simulink model "ExoskeletonControlModel"  (R2022b)
settings: Solver=ode3  StartTime=0.0  StopTime=inf  FixedStep=Ts  RelTol=1e-3
PreLoadFcn:
  | Ts_IO204 = 0.001;
  | 
  | if ~exist('Ts', 'var')
  | Ts = 0.001;
  | end
  | if ~exist('FPGA_Frequency', 'var')
  | FPGA_Frequency = 75000000;
  | end
  | 
  | ts_IO612 = 1e-3;
  | 
  | load('TargetReached.mat')
  | load('ActualPos_inc.mat')
model workspace (MAT data in the model file):
  DeltaData : timeseries (value not decoded)
  EC45_deg2incs = 2276
  EC60_deg2inc = 5461
  EC90_deg2incs = 7111
  Enc2rad_18bit = 2.3968e-05
  Enc2rad_19bit = 1.1984e-05
  Enc2rad_20bit = 5.9921e-06
  GiulioModel : robotics.RigidBodyTree (value not decoded)
  Giulio_Spheric_model : robotics.RigidBodyTree (value not decoded)
  Offset1_ticks = 571315
  Offset2_ticks = 590938.9928
  Offset3_ticks = 457912.8279
  Offset4_ticks = 482293.9763
  Offset5_ticks = 598735.9316
  Offset_M1 = 1.12645499896
  Offset_M2 = 4.02728553608
  Offset_M3 = 5.48587511336
  Offset_M4 = 2.03717511516
  Offset_M5 = 4.4996674016
  T1_Nm : object (value not decoded)
  T2_Nm : object (value not decoded)
  TBmodel : robotics.RigidBodyTree (value not decoded)
  Ts = 0.002
  Xg : object (value not decoded)
  Yg : object (value not decoded)
  Zg : object (value not decoded)
  a2 = 0.27
  change_variable = 0
  d1 = [0 0 0 0 0 0 0 0 0 0 0 0 ... (30001 elements, 30001x1)]
  d1_1 = 0.21074
  d2 = [0 0 0 0 0 0 0 0 0 0 0 0 ... (30001 elements, 30001x1)]
  d2_1 = 0.04864
  d3 = [0 0 0 0 0 0 0 0 0 0 0 0 ... (30001 elements, 30001x1)]
  d4 = [0 0 0 0 0 0 0 0 0 0 0 0 ... (30001 elements, 30001x1)]
  d5 = [0 0 0 0 0 0 0 0 0 0 0 0 ... (30001 elements, 30001x1)]
  d6 = [0 0 0 0 0 0 0 0 0 0 0 0 ... (30001 elements, 30001x1)]
  ee_x = -0.2852
  ee_y = -0.3683
  ee_z = -0.0386
  enc2rad_EC45 = 7.6699e-06
  enc2rad_EC90 = 2.3969e-05
  k1_Nm_ticks = 0.00923
  k2_Nm_ticks = 0.0257
  k3_Nm_ticks = 0.00692
  k4_Nm_ticks = 0.00729
  k5_Nm_ticks = 0.00641
  lower_lim_m1 = -330000
  lower_lim_m2 = -235302
  lower_lim_m3 = -132865
  lower_lim_m4 = -152732
  lower_lim_m5 = -138363
  lower_lim_m6 = -200325
  m1 = 2.441408578
  m2 = 3.750007
  m3 = 1.56250298
  m4 = 1.56250298
  m5 = 1.56250298
  m6 = 1.56250298
  n_oversampling = 8
  offset_sea_1 = 0.5547
  offset_sea_2 = 2.8595
  offset_sea_3 = 3.5058
  offset_sea_4 = 2.8586
  offset_sea_5 = 2.8736
  params : AKSIM (value not decoded)
  pos_th_neg = -180000
  pos_th_pos = 180000
  q1 = -1819347
  q2 = -196752
  q3 = -596465
  q4 = -556807
  q5 = -573932
  q6 = -489063
  sine = [0 0.187999937334 0.751998997352 1.69199492401 3.0079839574 4.6999608335 6.76791878442 9.21184953835 12.0317433196 15.2275888485 18.7993733417 22.7470825122 ... (12501 elements, 12501x1)]
  start : object (value not decoded)
  switch_admittance = 1
  t1 : object (value not decoded)
  t2 : object (value not decoded)
  torsionalStiffnes_M1 = 384.88
  torsionalStiffnes_M2 = 1500
  torsionalStiffnes_M3 = 901.97
  torsionalStiffnes_M4 = 950.86
  torsionalStiffnes_M5 = 930
  torsionalStiffnes_M6 = 914
  upper_lim_m1 = 340000
  upper_lim_m2 = 95467
  upper_lim_m3 = 164951
  upper_lim_m4 = 210607
  upper_lim_m5 = 252595
  upper_lim_m6 = 96694
  vel_th_neg = -100
  vel_th_pos = 100
  x = 0
undefined symbols (not defined in the file): C, DiscIntNeverNeededParam
libraries: canmsglib x285, speedgoatlib_IO614 x245, simulink x26, slrealtimeloglib x9, simulink_extras x6, robotmaniplib x6
(part 9 of 13)

== system ExoskeletonControlModel/OutputDataTX/TX_EPOS4_M3_M5/rxSDO4 ==
  Trigger : TriggerPort  VariantControl=Variant  PortDimensions=1
  CAN Write : speedgoatlib_IO614/CAN/CAN Write  id=1  sampleTime=-1  portSelection=4  messageType=CAN  enaStatusPort=off  protl=IO614  ptIdx=3  isFDMod=0
  CS : Constant  Value=hex2dec('40')
  Index : Constant  Value=hex2dec('3012')
  ParamData : Constant  Value=hex2dec('000F')
  Subindex : Constant  Value=hex2dec('09')
  rxSDO : canmsglib/CAN Pack  MsgList=(none)  MsgName=CAN Msg  MsgIDType=Standard (11-bit identifier)  MsgIdentifier=1540  MsgLength=8  Remote=off  ApplyMinMax=off  BusOutput=off  SignalInfo={ 'CS', '0', '8', 'LE', 'unsigned', 'Standard', '0', '1', '0', '-Inf', 'Inf'; 'Index', '8', '16', 'LE', 'unsigned', 'Standard', '0', '1', '0', '-Inf', 'Inf'; 'SubIndex', '24', '8', 'LE', 'unsigned', 'Standard', '0', '1', '0', '-Inf', 'Inf'; 'ParamData', '32', '32', 'LE', 'signed', 'Standard', '0', '1', '0', '-Inf', 'Inf' }
      settings: DataFormat=manually specified signals
  wires:
  rxSDO/1 -> CAN Write/1
  CS/1 -> rxSDO/1
  Index/1 -> rxSDO/2
  Subindex/1 -> rxSDO/3
  ParamData/1 -> rxSDO/4

== system ExoskeletonControlModel/OutputDataTX/TX_EPOS4_M3_M5/set_NMT_state ==
  Input : Inport
  Trigger : TriggerPort  VariantControl=Variant  PortDimensions=1
  CAN Write : speedgoatlib_IO614/CAN/CAN Write  id=1  sampleTime=-1  portSelection=4  messageType=CAN  enaStatusPort=off  protl=IO614  ptIdx=3  isFDMod=0
  NodeID : Constant  Value=0
  set_NMT_state : canmsglib/CAN Pack  MsgList=(none)  MsgName=CAN Msg  MsgIDType=Standard (11-bit identifier)  MsgIdentifier=0  MsgLength=2  Remote=off  ApplyMinMax=off  BusOutput=off  SignalInfo={ 'CS', '0', '8', 'LE', 'unsigned', 'Standard', '0', '1', '0', '-Inf', 'Inf'; 'NodeID', '8', '8', 'LE', 'unsigned', 'Standard', '0', '1', '0', '-Inf', 'Inf' }
      settings: DataFormat=manually specified signals
  wires:
  Input/1 -> set_NMT_state/1
  NodeID/1 -> set_NMT_state/2
  set_NMT_state/1 -> CAN Write/1

== system ExoskeletonControlModel/DataProcessing/CST_trasparency/CST_control/MOTOR3 ==
  note: FrictionCompensation
  note: IMPEDENCE CONTROL M3
  note: CURRENT CONTROL M3
  TauSEA : Inport
  Gravity : Inport  Port=2
  position : Inport  Port=3
  speed_rads : Inport  Port=4
  State : Inport  Port=5
  MovLenght : Inport  Port=6
  Reset : Inport  Port=7
  Enable : EnablePort
  Abs : Abs  SaturateOnIntegerOverflow=off
  Chart : Stateflow chart  TreatAsAtomicUnit=on
  Constant1 : Constant  Value=-0.1
  Data Store Read : DataStoreRead  DataStoreName=Start_m3  IndexOptions=Index vector (dialog)  Indices=1  OutputSizes=1
  Data Store Read2 : DataStoreRead  DataStoreName=Spring_m3  IndexOptions=Index vector (dialog)  Indices=1  OutputSizes=1
  Degrees to Radians : simulink_extras/Transformations/Degrees to Radians
  Delay1 : Delay  DelayLength=1
  Enc2rad : Gain  Gain=1/(2276)
  Gain : Gain  Gain=1/100
  Gain1 : Gain  Gain=9.5492965964254
  Product : Product
  Product2 : Product
  Product3 : Product
  Subsystem1 : Subsystem
  Sum : Sum  Inputs=|++
  Sum2 : Sum  Inputs=|-+
  Sum3 : Sum  Inputs=|++
  Sum4 : Sum  Inputs=|+-
  Sum5 : Sum  Inputs=++++
  Terminator : Terminator
  Terminator1 : Terminator
  Thousands of nominal torque EC2 : Gain  Gain=8442.5
  impedance_values_safe_zones : Stateflow chart  TreatAsAtomicUnit=on
  Reference Drive Current | Volt1 : Outport
  SignalEnded3 : Outport  Port=2  InitialOutput=0
  LeR_M3 : Outport  Port=3  InitialOutput=0
  wires:
  Sum5/1 -> Product/2
  Enc2rad/1 -> Degrees to Radians/1  "DeltaPos_rad"
  Sum4/1 -> Enc2rad/1  "DeltaPos_inc"
  impedance_values_safe_zones/1(new_target_torque) -> Sum5/3
  Subsystem1/1(RefPosLR) -> LeR_M3/1, Sum4/1
  Gravity/1 -> Sum/2, Sum5/1
  impedance_values_safe_zones/2(y) -> Terminator1/1
  Sum3/1 -> Sum/1, impedance_values_safe_zones/1(torque)
  Constant1/1 -> Sum3/2
  Degrees to Radians/1 -> Product2/1
  TauSEA/1 -> Sum3/1
  Data Store Read2/1 -> Product2/2
  Data Store Read/1 -> Product/1
  position/1 -> impedance_values_safe_zones/2(theta), Sum4/2
  Product/1 -> Thousands of nominal torque EC2/1
  Thousands of nominal torque EC2/1 -> Gain/1  "Reference Drive Current | Volt"
  Sum/1 -> Sum5/2
  Gain/1 -> Reference Drive Current | Volt1/1
  speed_rads/1 -> Gain1/1, Product3/2, impedance_values_safe_zones/3(speed)
  Chart/1(beta) -> Product3/1
  Abs/1 -> Chart/2(speed)
  State/1 -> Chart/1(state)
  Gain1/1 -> Abs/1
  Sum2/1 -> Sum5/4
  Product3/1 -> Sum2/1
  MovLenght/1 -> Subsystem1/2(sz)
  Reset/1 -> Subsystem1/Enable, Delay1/1
  Delay1/1 -> Subsystem1/1(In1)
  Subsystem1/3(Out2) -> Terminator/1
  Subsystem1/2(signal_ended) -> SignalEnded3/1
  Product2/1 -> Sum2/2

== system ExoskeletonControlModel/DataProcessing/CST_trasparency/CST_control/MOTOR4 ==
  note: CURRENT CONTROL M4
  note: IMPEDENCE CONTROL M4
  note: FrictionCompensation
  TauSEA : Inport
  Gravity : Inport  Port=2
  position : Inport  Port=3
  speed_rads : Inport  Port=4
  In6 : Inport  Port=5
  MovLenght : Inport  Port=6
  Reset : Inport  Port=7
  Enable : EnablePort
  Abs : Abs  SaturateOnIntegerOverflow=off
  Chart : Stateflow chart  TreatAsAtomicUnit=on
  Constant : Constant  Value=-0.1
  Data Store Read : DataStoreRead  DataStoreName=Start_m4  IndexOptions=Index vector (dialog)  Indices=1  OutputSizes=1
  Data Store Read2 : DataStoreRead  DataStoreName=Spring_m4  IndexOptions=Index vector (dialog)  Indices=1  OutputSizes=1
  Degrees to Radians : simulink_extras/Transformations/Degrees to Radians
  Delay1 : Delay  DelayLength=1
  Enc2rad : Gain  Gain=1/(2276)
  Gain : Gain  Gain=1/100
  Gain1 : Gain  Gain=9.5492965964254
  Product : Product
  Product2 : Product
  Product3 : Product
  Subsystem1 : Subsystem
  Sum : Sum  Inputs=|++
  Sum2 : Sum  Inputs=|++
  Sum3 : Sum  Inputs=|+-
  Sum4 : Sum  Inputs=++++
  Sum5 : Sum  Inputs=|-+
  Terminator : Terminator
  Terminator1 : Terminator
  Thousands of nominal torque EC2 : Gain  Gain=8442.5
  impedance_values_safe_zones : Stateflow chart  TreatAsAtomicUnit=on
  Reference Drive Current | Volt1 : Outport
  SignalEnded3 : Outport  Port=2
  LeR_M4 : Outport  Port=3
  wires:
  Constant/1 -> Sum2/2
  impedance_values_safe_zones/2(y) -> Terminator1/1
  Gravity/1 -> Sum/1, Sum4/1
  position/1 -> impedance_values_safe_zones/2(theta), Sum3/2
  Data Store Read/1 -> Product/1
  impedance_values_safe_zones/1(new_target_torque) -> Sum4/3
  Product2/1 -> Sum5/2
  Sum3/1 -> Enc2rad/1  "DeltaPos_inc"
  Degrees to Radians/1 -> Product2/1
  Subsystem1/1(RefPosLR) -> LeR_M4/1, Sum3/1
  Sum4/1 -> Product/2
  Enc2rad/1 -> Degrees to Radians/1  "DeltaPos_rad"
  TauSEA/1 -> Sum2/1
  Sum2/1 -> Sum/2, impedance_values_safe_zones/1(torque)
  Data Store Read2/1 -> Product2/2
  Product/1 -> Thousands of nominal torque EC2/1
  Thousands of nominal torque EC2/1 -> Gain/1  "Reference Drive Current | Volt"
  Gain/1 -> Reference Drive Current | Volt1/1
  Sum/1 -> Sum4/2
  Chart/1(beta) -> Product3/1
  Gain1/1 -> Abs/1
  speed_rads/1 -> Product3/2, Gain1/1, impedance_values_safe_zones/3(speed)
  Product3/1 -> Sum5/1
  In6/1 -> Chart/1(state)
  Abs/1 -> Chart/2(speed)
  Sum5/1 -> Sum4/4
  Subsystem1/3(Out2) -> Terminator/1
  MovLenght/1 -> Subsystem1/2(sz)
  Delay1/1 -> Subsystem1/1(In1)
  Reset/1 -> Delay1/1, Subsystem1/Enable
  Subsystem1/2(signal_ended) -> SignalEnded3/1

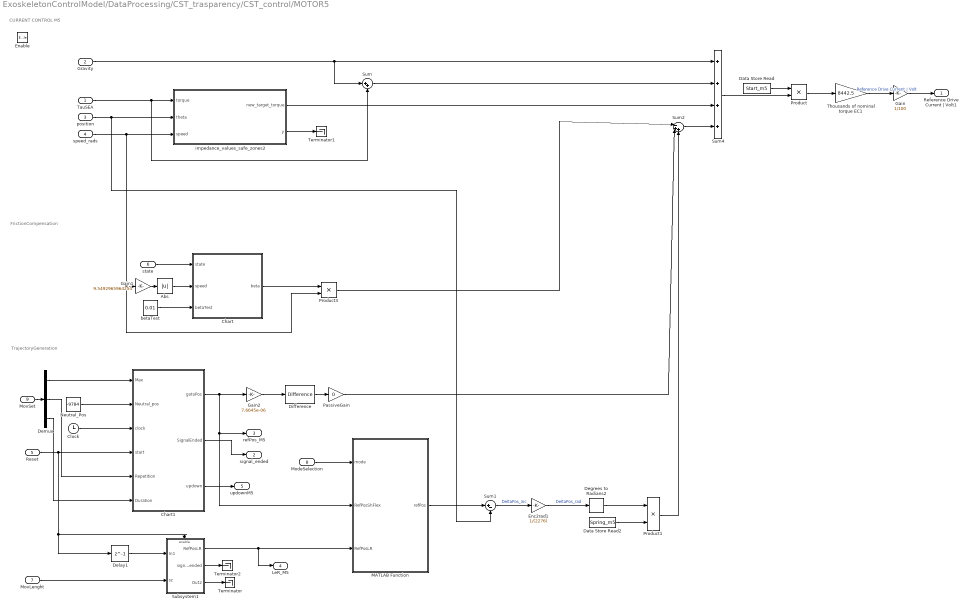
== system ExoskeletonControlModel/DataProcessing/CST_trasparency/CST_control/MOTOR5 ==
  note: TrajectoryGeneration
  note: CURRENT CONTROL M5
  note: FrictionCompensation
  TauSEA : Inport
  Gravity : Inport  Port=2
  position : Inport  Port=3
  speed_rads : Inport  Port=4
  Reset : Inport  Port=5
  state : Inport  Port=6
  MovLenght : Inport  Port=7
  ModeSelection : Inport  Port=8
  MovSet : Inport  Port=9
  Enable : EnablePort
  Abs : Abs  SaturateOnIntegerOverflow=off
  Chart : Stateflow chart  TreatAsAtomicUnit=on
  Chart1 : Stateflow chart  TreatAsAtomicUnit=on
  Clock : Clock
      settings: Decimation=1000
  Data Store Read : DataStoreRead  DataStoreName=Start_m5  IndexOptions=Index vector (dialog)  Indices=1  OutputSizes=1
  Data Store Read2 : DataStoreRead  DataStoreName=Spring_m5  IndexOptions=Index vector (dialog)  Indices=1  OutputSizes=1
  Degrees to Radians2 : simulink_extras/Transformations/Degrees to Radians
  Delay1 : Delay  DelayLength=1
  Demux : Demux  Outputs=3
  Difference : simulink/Discrete/Difference  ICPrevInput=0.0  OutMin=[]  OutMax=[]  OutDataType=fixdt(1, 16)  OutScaling=2^-10  DoSatur=off
  Enc2rad1 : Gain  Gain=1/(2276)
  Gain : Gain  Gain=1/100
  Gain1 : Gain  Gain=9.5492965964254
  Gain2 : Gain  Gain=7.6645e-06
  MATLAB Function : MATLAB Function  TreatAsAtomicUnit=on
  Neutral_Pos : Constant  Value=-9784
  PassiveGain : Gain  Gain=0
  Product : Product
  Product1 : Product
  Product3 : Product
  Subsystem1 : Subsystem
  Sum : Sum  Inputs=|++
  Sum1 : Sum  Inputs=|+-
  Sum2 : Sum  Inputs=|-++
  Sum4 : Sum  Inputs=++++
  Terminator : Terminator
  Terminator1 : Terminator
  Terminator2 : Terminator
  Thousands of nominal torque EC1 : Gain  Gain=8442.5
  betaTest : Constant  Value=0.01
  impedance_values_safe_zones2 : Stateflow chart  TreatAsAtomicUnit=on
  Reference Drive Current | Volt1 : Outport
  signal_ended : Outport  Port=2  InitialOutput=0
  refPos_M5 : Outport  Port=3
  LeR_M5 : Outport  Port=4
  updownM5 : Outport  Port=5  InitialOutput=0
  wires:
  impedance_values_safe_zones2/1(new_target_torque) -> Sum4/3
  Sum4/1 -> Product/2
  Gravity/1 -> Sum/1, Sum4/1
  Thousands of nominal torque EC1/1 -> Gain/1  "Reference Drive Current | Volt"
  TauSEA/1 -> Sum/2, impedance_values_safe_zones2/1(torque)
  impedance_values_safe_zones2/2(y) -> Terminator1/1
  Data Store Read/1 -> Product/1
  Product3/1 -> Sum2/1
  speed_rads/1 -> impedance_values_safe_zones2/3(speed), Gain1/1, Product3/2
  position/1 -> impedance_values_safe_zones2/2(theta), Sum1/2
  Sum2/1 -> Sum4/4
  Sum/1 -> Sum4/2
  Gain/1 -> Reference Drive Current | Volt1/1
  Product/1 -> Thousands of nominal torque EC1/1
  Abs/1 -> Chart/2(speed)
  Gain1/1 -> Abs/1
  state/1 -> Chart/1(state)
  Product1/1 -> Sum2/3
  Neutral_Pos/1 -> Chart1/2(Neutral_pos)
  Chart1/1(gotoPos) -> refPos_M5/1, MATLAB Function/2(RefPosShFlex), Gain2/1
  Clock/1 -> Chart1/3(clock)
  Chart1/2(SignalEnded) -> signal_ended/1
  Data Store Read2/1 -> Product1/2
  Sum1/1 -> Enc2rad1/1  "DeltaPos_inc"
  Enc2rad1/1 -> Degrees to Radians2/1  "DeltaPos_rad"
  Degrees to Radians2/1 -> Product1/1
  Gain2/1 -> Difference/1
  Difference/1 -> PassiveGain/1
  PassiveGain/1 -> Sum2/2
  Delay1/1 -> Subsystem1/1(In1)
  MovLenght/1 -> Subsystem1/2(sz)
  Reset/1 -> Subsystem1/Enable, Delay1/1, Chart1/4(start)
  ModeSelection/1 -> MATLAB Function/1(mode)
  MATLAB Function/1(refPos) -> Sum1/1
  Subsystem1/1(RefPosLR) -> LeR_M5/1, MATLAB Function/3(RefPosLR)
  Subsystem1/3(Out2) -> Terminator/1
  Subsystem1/2(signal_ended) -> Terminator2/1
  Chart/1(beta) -> Product3/1
  betaTest/1 -> Chart/3(betaTest)
  Chart1/3(updown) -> updownM5/1
  Demux/1 -> Chart1/1(Max)
  Demux/2 -> Chart1/5(Repetition)
  Demux/3 -> Chart1/6(Duration)
  MovSet/1 -> Demux/1

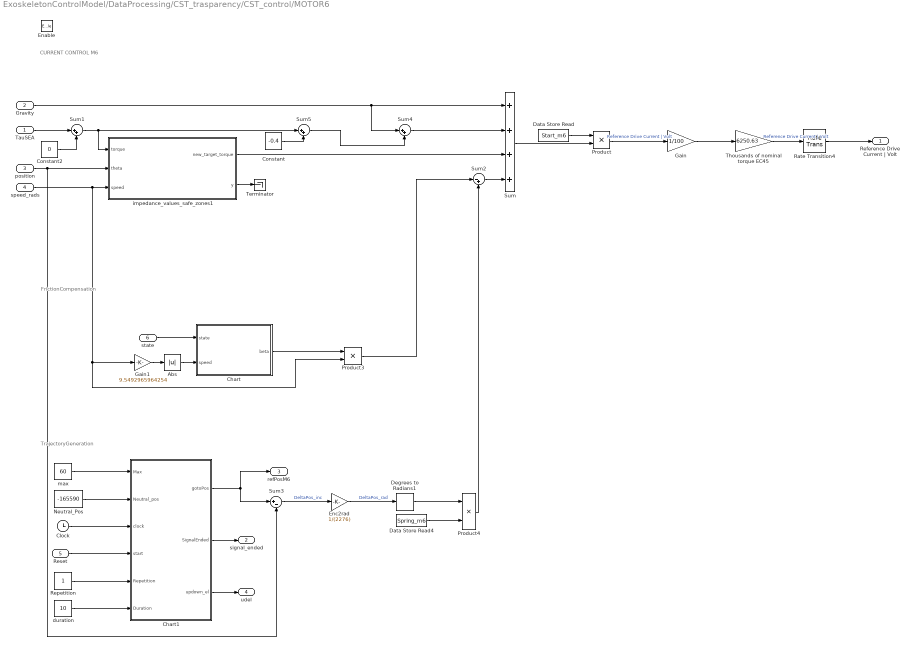
== system ExoskeletonControlModel/DataProcessing/CST_trasparency/CST_control/MOTOR6 ==
  note: TrajectoryGeneration
  note: CURRENT CONTROL M6
  note: FrictionCompensation
  TauSEA : Inport
  Gravity : Inport  Port=2
  position : Inport  Port=3
  speed_rads : Inport  Port=4
  Reset : Inport  Port=5
  state : Inport  Port=6
  Enable : EnablePort
  Abs : Abs  SaturateOnIntegerOverflow=off
  Chart : Stateflow chart  TreatAsAtomicUnit=on
  Chart1 : Stateflow chart  TreatAsAtomicUnit=on
  Clock : Clock
      settings: Decimation=1000
  Constant : Constant  Value=-0.4
  Constant2 : Constant  Value=0
  Data Store Read : DataStoreRead  DataStoreName=Start_m6  IndexOptions=Index vector (dialog)  Indices=1  OutputSizes=1
  Data Store Read4 : DataStoreRead  DataStoreName=Spring_m6  IndexOptions=Index vector (dialog)  Indices=1  OutputSizes=1
  Degrees to Radians1 : simulink_extras/Transformations/Degrees to Radians
  Enc2rad : Gain  Gain=1/(2276)
  Gain : Gain  Gain=1/100
  Gain1 : Gain  Gain=9.5492965964254
  Neutral_Pos : Constant  Value=-165590
  Product : Product
  Product3 : Product
  Product4 : Product
  Rate Transition4 : RateTransition  Deterministic=off  OutPortSampleTime=Ts
  Repetition : Constant
  Sum : Sum  Inputs=++++
  Sum1 : Sum  Inputs=|++
  Sum2 : Sum  Inputs=|-+
  Sum3 : Sum  Inputs=|+-
  Sum4 : Sum  Inputs=|++
  Sum5 : Sum  Inputs=|++
  Terminator : Terminator
  Thousands of nominal torque EC45 : Gain  Gain=6250.63
  duration : Constant  Value=10
  impedance_values_safe_zones1 : Stateflow chart  TreatAsAtomicUnit=on
  max : Constant  Value=60
  Reference Drive Current | Volt : Outport
  signal_ended : Outport  Port=2  InitialOutput=0
  refPosM6 : Outport  Port=3
  udel : Outport  Port=4  InitialOutput=0
  wires:
  Sum/1 -> Product/2
  impedance_values_safe_zones1/1(new_target_torque) -> Sum/3
  Reset/1 -> Chart1/4(start)
  impedance_values_safe_zones1/2(y) -> Terminator/1
  Data Store Read/1 -> Product/1
  speed_rads/1 -> Product3/2, Gain1/1, impedance_values_safe_zones1/3(speed)
  position/1 -> impedance_values_safe_zones1/2(theta), Sum3/2
  Sum3/1 -> Enc2rad/1  "DeltaPos_inc"
  Sum2/1 -> Sum/4
  Product3/1 -> Sum2/1
  Enc2rad/1 -> Degrees to Radians1/1  "DeltaPos_rad"
  Product4/1 -> Sum2/2
  Data Store Read4/1 -> Product4/2
  Degrees to Radians1/1 -> Product4/1
  Chart/1(beta) -> Product3/1
  Sum1/1 -> Sum5/1, impedance_values_safe_zones1/1(torque)
  TauSEA/1 -> Sum1/1
  Constant2/1 -> Sum1/2
  Rate Transition4/1 -> Reference Drive Current | Volt/1
  Product/1 -> Gain/1  "Reference Drive Current | Volt"
  Gain/1 -> Thousands of nominal torque EC45/1
  Thousands of nominal torque EC45/1 -> Rate Transition4/1  "Reference Drive Current | Volt"
  Gravity/1 -> Sum4/1, Sum/1
  Sum4/1 -> Sum/2
  Constant/1 -> Sum5/2
  Sum5/1 -> Sum4/2
  state/1 -> Chart/1(state)
  Gain1/1 -> Abs/1
  Abs/1 -> Chart/2(speed)
  Repetition/1 -> Chart1/5(Repetition)
  Clock/1 -> Chart1/3(clock)
  Chart1/2(SignalEnded) -> signal_ended/1
  duration/1 -> Chart1/6(Duration)
  Neutral_Pos/1 -> Chart1/2(Neutral_pos)
  max/1 -> Chart1/1(Max)
  Chart1/1(gotoPos) -> Sum3/1, refPosM6/1
  Chart1/3(updown_el) -> udel/1

== system ExoskeletonControlModel/DataProcessing/CST_trasparency/CST_control/SendPositionToEPOS ==
  note: SEND TARGET POSITION TO EPOS SERVOMOTOR CONTROLLER
  PosM5 : Inport
  Enable : EnablePort
  Constant : Constant  Value=-165590
  receive_PDO3_m5 : Subsystem
  receive_PDO3_m6 : Subsystem
  wires:
  PosM5/1 -> receive_PDO3_m5/1(target_pos)  "PositionCommandEPOSM5_inc"
  Constant/1 -> receive_PDO3_m6/1(target_pos)  "PositionCommandEPOSM6_inc"

== system ExoskeletonControlModel/DataProcessing/CST_trasparency/CST_control/SendPositionToEPOS1 ==
  note: SEND TARGET POSITION TO EPOS SERVOMOTOR CONTROLLER
  PosM6 : Inport
  Enable : EnablePort
  Constant : Constant  Value=-9784
  receive_PDO3_m5 : Subsystem
  receive_PDO3_m6 : Subsystem
  wires:
  Constant/1 -> receive_PDO3_m5/1(target_pos)  "PositionCommandEPOSM5_inc"
  PosM6/1 -> receive_PDO3_m6/1(target_pos)  "PositionCommandEPOSM6_inc"

== system ExoskeletonControlModel/DataProcessing/CST_trasparency/CST_control/SendPositionToEPOS2 ==
  note: SEND TARGET POSITION TO EPOS SERVOMOTOR CONTROLLER
  PosM3 : Inport
  PosM4 : Inport  Port=2
  PosM5 : Inport  Port=3
  Enable : EnablePort
  receive_PDO3_m1 : Subsystem
  receive_PDO3_m5 : Subsystem
  receive_PDO3_m6 : Subsystem
  wires:
  PosM5/1 -> receive_PDO3_m5/1(target_pos)  "PositionCommandEPOSM5_inc"
  PosM3/1 -> receive_PDO3_m6/1(target_pos)  "PositionCommandEPOSM6_inc"
  PosM4/1 -> receive_PDO3_m1/1(target_pos)  "PositionCommandEPOSM5_inc"

== system ExoskeletonControlModel/DataProcessing/CST_trasparency/SendTorqueCommand/Subsystem ==
  TAU_M6 : Inport
  Enable : EnablePort
  Bus Creator7 : BusCreator  Inputs=3
  receive_PDO4_m6 : Subsystem
  target_velocity_m6 : Constant  Value=0  SampleTime=-1
  torque_offset_m6 : Constant  Value=0  SampleTime=-1
  wires:
  torque_offset_m6/1 -> Bus Creator7/3  "torque_offset_m6"
  TAU_M6/1 -> Bus Creator7/2
  target_velocity_m6/1 -> Bus Creator7/1  "target_velocity_m6"
  Bus Creator7/1 -> receive_PDO4_m6/1(velocity_torque_offset)

== system ExoskeletonControlModel/DataProcessing/CST_trasparency/SendTorqueCommand/Subsystem1 ==
  TAU_M4 : Inport
  Enable : EnablePort
  Bus Creator1 : BusCreator  Inputs=3
  receive_PDO4_m4 : Subsystem
  target_velocity_m4 : Constant  Value=0
  torque_offset_m4 : Constant  Value=0
  wires:
  Bus Creator1/1 -> receive_PDO4_m4/1(velocity_torque_offset)
  torque_offset_m4/1 -> Bus Creator1/3  "torque_offset_m4"
  target_velocity_m4/1 -> Bus Creator1/1  "target_velocity_m4"
  TAU_M4/1 -> Bus Creator1/2

== system ExoskeletonControlModel/DataProcessing/CST_trasparency/SendTorqueCommand/Subsystem2 ==
  TAU_M5 : Inport
  Enable : EnablePort
  Bus Creator2 : BusCreator  Inputs=3
  receive_PDO4_m5 : Subsystem
  target_velocity_m5 : Constant  Value=0
  torque_offset_m5 : Constant  Value=0
  wires:
  TAU_M5/1 -> Bus Creator2/2
  target_velocity_m5/1 -> Bus Creator2/1  "target_velocity_m5"
  Bus Creator2/1 -> receive_PDO4_m5/1(velocity_torque_offset)
  torque_offset_m5/1 -> Bus Creator2/3  "torque_offset_m5"

== system ExoskeletonControlModel/DataProcessing/CST_trasparency/SendTorqueCommand/Subsystem3 ==
  TAU_M3 : Inport
  Enable : EnablePort
  Bus Creator : BusCreator  Inputs=3
  receive_PDO4_m3 : Subsystem
  target_velocity_m3 : Constant  Value=0
  torque_offset_m3 : Constant  Value=0
  wires:
  TAU_M3/1 -> Bus Creator/2
  Bus Creator/1 -> receive_PDO4_m3/1(velocity_torque_offset)
  target_velocity_m3/1 -> Bus Creator/1  "target_velocity_m3"
  torque_offset_m3/1 -> Bus Creator/3  "torque_offset_m3"

== system ExoskeletonControlModel/DataProcessing/CST_trasparency/SendTorqueCommand/Subsystem4 ==
  target_torque_m1 : Inport
  Enable : EnablePort
  Bus Creator : BusCreator  Inputs=3
  receive_PDO4_m1 : Subsystem
  target_velocity_m1 : Constant  Value=0
  torque_offset_m1 : Constant  Value=0
  wires:
  target_velocity_m1/1 -> Bus Creator/1  "target_velocity_m1"
  Bus Creator/1 -> receive_PDO4_m1/1(velocity_torque_offset)
  torque_offset_m1/1 -> Bus Creator/3  "torque_offset_m1"
  target_torque_m1/1 -> Bus Creator/2

== system ExoskeletonControlModel/DataProcessing/Homing_State_Machine/Homing_m1/FAULT.Fault_reset/receive_PDO1_m1 ==
  controlword : Inport
  CAN Write : speedgoatlib_IO614/CAN/CAN Write  id=1  sampleTime=-1  portSelection=3  messageType=CAN  enaStatusPort=off  protl=IO614  ptIdx=2  isFDMod=0
  set_controlword : canmsglib/CAN Pack  MsgList=(none)  MsgName=CAN Msg  MsgIDType=Standard (11-bit identifier)  MsgIdentifier=hex2dec('201')  MsgLength=2  Remote=off  ApplyMinMax=off  BusOutput=off  SignalInfo={ 'controlword', '0', '16', 'LE', 'unsigned', 'Standard', '0', '1', '0', '-Inf', 'Inf' }
      settings: DataFormat=manually specified signals
  wires:
  controlword/1 -> set_controlword/1
  set_controlword/1 -> CAN Write/1

== system ExoskeletonControlModel/DataProcessing/Homing_State_Machine/Homing_m1/FAULT.ST4_shutdown/receive_PDO1_m1 ==
  controlword : Inport
  CAN Write : speedgoatlib_IO614/CAN/CAN Write  id=1  sampleTime=-1  portSelection=3  messageType=CAN  enaStatusPort=off  protl=IO614  ptIdx=2  isFDMod=0
  set_controlword : canmsglib/CAN Pack  MsgList=(none)  MsgName=CAN Msg  MsgIDType=Standard (11-bit identifier)  MsgIdentifier=hex2dec('201')  MsgLength=2  Remote=off  ApplyMinMax=off  BusOutput=off  SignalInfo={ 'controlword', '0', '16', 'LE', 'unsigned', 'Standard', '0', '1', '0', '-Inf', 'Inf' }
      settings: DataFormat=manually specified signals
  wires:
  controlword/1 -> set_controlword/1
  set_controlword/1 -> CAN Write/1

== system ExoskeletonControlModel/DataProcessing/Homing_State_Machine/Homing_m1/HOMING.ST10_set_PPM/receive_PDO2_m1 ==
  mode : Inport
  Bus Selector : BusSelector  OutputSignals=mode_m1,interpolation_period_m1
  CAN Write : speedgoatlib_IO614/CAN/CAN Write  id=1  sampleTime=-1  portSelection=3  messageType=CAN  enaStatusPort=off  protl=IO614  ptIdx=2  isFDMod=0
  set_mode : canmsglib/CAN Pack  MsgList=(none)  MsgName=CAN Msg  MsgIDType=Standard (11-bit identifier)  MsgIdentifier=hex2dec('301')  MsgLength=2  Remote=off  ApplyMinMax=off  BusOutput=off  SignalInfo={ 'mode', '0', '8', 'LE', 'unsigned', 'Standard', '0', '1', '0', '-Inf', 'Inf'; 'interpolation time period', '8', '8', 'LE', 'unsigned', 'Standard', '0', '1', '0', '-Inf', 'Inf' }
      settings: DataFormat=manually specified signals
  wires:
  set_mode/1 -> CAN Write/1
  mode/1 -> Bus Selector/1
  Bus Selector/1 -> set_mode/1  "<mode_m1>"
  Bus Selector/2 -> set_mode/2  "<interpolation_period_m1>"

== system ExoskeletonControlModel/DataProcessing/Homing_State_Machine/Homing_m1/HOMING.ST11_shutdown1/receive_PDO1_m1 ==
  controlword : Inport
  CAN Write : speedgoatlib_IO614/CAN/CAN Write  id=1  sampleTime=-1  portSelection=3  messageType=CAN  enaStatusPort=off  protl=IO614  ptIdx=2  isFDMod=0
  set_controlword : canmsglib/CAN Pack  MsgList=(none)  MsgName=CAN Msg  MsgIDType=Standard (11-bit identifier)  MsgIdentifier=hex2dec('201')  MsgLength=2  Remote=off  ApplyMinMax=off  BusOutput=off  SignalInfo={ 'controlword', '0', '16', 'LE', 'unsigned', 'Standard', '0', '1', '0', '-Inf', 'Inf' }
      settings: DataFormat=manually specified signals
  wires:
  controlword/1 -> set_controlword/1
  set_controlword/1 -> CAN Write/1

== system ExoskeletonControlModel/DataProcessing/Homing_State_Machine/Homing_m1/HOMING.ST12_Switch_on_and_Enable_Operation/receive_PDO1_m1 ==
  controlword : Inport
  CAN Write : speedgoatlib_IO614/CAN/CAN Write  id=1  sampleTime=-1  portSelection=3  messageType=CAN  enaStatusPort=off  protl=IO614  ptIdx=2  isFDMod=0
  set_controlword : canmsglib/CAN Pack  MsgList=(none)  MsgName=CAN Msg  MsgIDType=Standard (11-bit identifier)  MsgIdentifier=hex2dec('201')  MsgLength=2  Remote=off  ApplyMinMax=off  BusOutput=off  SignalInfo={ 'controlword', '0', '16', 'LE', 'unsigned', 'Standard', '0', '1', '0', '-Inf', 'Inf' }
      settings: DataFormat=manually specified signals
  wires:
  controlword/1 -> set_controlword/1
  set_controlword/1 -> CAN Write/1

== system ExoskeletonControlModel/DataProcessing/Homing_State_Machine/Homing_m1/HOMING.ST13_send_target_pos/receive_PDO3_m1 ==
  target_pos : Inport
  CAN Write : speedgoatlib_IO614/CAN/CAN Write  id=1  sampleTime=-1  portSelection=3  messageType=CAN  enaStatusPort=off  protl=IO614  ptIdx=2  isFDMod=0
  set_position : canmsglib/CAN Pack  MsgList=(none)  MsgName=CAN Msg  MsgIDType=Standard (11-bit identifier)  MsgIdentifier=hex2dec('401')  MsgLength=4  Remote=off  ApplyMinMax=off  BusOutput=off  SignalInfo={ 'target position', '0', '32', 'LE', 'signed', 'Standard', '0', '1', '0', '-Inf', 'Inf' }
      settings: DataFormat=manually specified signals
  wires:
  target_pos/1 -> set_position/1
  set_position/1 -> CAN Write/1

== system ExoskeletonControlModel/DataProcessing/Homing_State_Machine/Homing_m1/HOMING.ST14_Abs_ref_start_immediatly/receive_PDO1_m1 ==
  controlword : Inport
  CAN Write : speedgoatlib_IO614/CAN/CAN Write  id=1  sampleTime=-1  portSelection=3  messageType=CAN  enaStatusPort=off  protl=IO614  ptIdx=2  isFDMod=0
  set_controlword : canmsglib/CAN Pack  MsgList=(none)  MsgName=CAN Msg  MsgIDType=Standard (11-bit identifier)  MsgIdentifier=hex2dec('201')  MsgLength=2  Remote=off  ApplyMinMax=off  BusOutput=off  SignalInfo={ 'controlword', '0', '16', 'LE', 'unsigned', 'Standard', '0', '1', '0', '-Inf', 'Inf' }
      settings: DataFormat=manually specified signals
  wires:
  controlword/1 -> set_controlword/1
  set_controlword/1 -> CAN Write/1

== system ExoskeletonControlModel/DataProcessing/Homing_State_Machine/Homing_m1/HOMING.ST15_set_home_mode/receive_PDO2_m1 ==
  mode : Inport
  Bus Selector : BusSelector  OutputSignals=mode_m1,interpolation_period_m1
  CAN Write : speedgoatlib_IO614/CAN/CAN Write  id=1  sampleTime=-1  portSelection=3  messageType=CAN  enaStatusPort=off  protl=IO614  ptIdx=2  isFDMod=0
  set_mode : canmsglib/CAN Pack  MsgList=(none)  MsgName=CAN Msg  MsgIDType=Standard (11-bit identifier)  MsgIdentifier=hex2dec('301')  MsgLength=2  Remote=off  ApplyMinMax=off  BusOutput=off  SignalInfo={ 'mode', '0', '8', 'LE', 'unsigned', 'Standard', '0', '1', '0', '-Inf', 'Inf'; 'interpolation time period', '8', '8', 'LE', 'unsigned', 'Standard', '0', '1', '0', '-Inf', 'Inf' }
      settings: DataFormat=manually specified signals
  wires:
  set_mode/1 -> CAN Write/1
  mode/1 -> Bus Selector/1
  Bus Selector/1 -> set_mode/1  "<mode_m1>"
  Bus Selector/2 -> set_mode/2  "<interpolation_period_m1>"

== system ExoskeletonControlModel/DataProcessing/Homing_State_Machine/Homing_m1/HOMING.ST1_Enter_Pre_Operational/set_NMT_state ==
  Input : Inport
  CAN Write : speedgoatlib_IO614/CAN/CAN Write  id=1  sampleTime=-1  portSelection=3  messageType=CAN  enaStatusPort=off  protl=IO614  ptIdx=2  isFDMod=0
  NodeID : Constant  Value=0
  set_NMT_state : canmsglib/CAN Pack  MsgList=(none)  MsgName=CAN Msg  MsgIDType=Standard (11-bit identifier)  MsgIdentifier=0  MsgLength=2  Remote=off  ApplyMinMax=off  BusOutput=off  SignalInfo={ 'CS', '0', '8', 'LE', 'unsigned', 'Standard', '0', '1', '0', '-Inf', 'Inf'; 'NodeID', '8', '8', 'LE', 'unsigned', 'Standard', '0', '1', '0', '-Inf', 'Inf' }
      settings: DataFormat=manually specified signals
  wires:
  Input/1 -> set_NMT_state/1
  NodeID/1 -> set_NMT_state/2
  set_NMT_state/1 -> CAN Write/1

== system ExoskeletonControlModel/DataProcessing/Homing_State_Machine/Homing_m1/HOMING.ST2_operational/set_NMT_state ==
  Input : Inport
  CAN Write : speedgoatlib_IO614/CAN/CAN Write  id=1  sampleTime=-1  portSelection=3  messageType=CAN  enaStatusPort=off  protl=IO614  ptIdx=2  isFDMod=0
  NodeID : Constant  Value=0
  set_NMT_state : canmsglib/CAN Pack  MsgList=(none)  MsgName=CAN Msg  MsgIDType=Standard (11-bit identifier)  MsgIdentifier=0  MsgLength=2  Remote=off  ApplyMinMax=off  BusOutput=off  SignalInfo={ 'CS', '0', '8', 'LE', 'unsigned', 'Standard', '0', '1', '0', '-Inf', 'Inf'; 'NodeID', '8', '8', 'LE', 'unsigned', 'Standard', '0', '1', '0', '-Inf', 'Inf' }
      settings: DataFormat=manually specified signals
  wires:
  Input/1 -> set_NMT_state/1
  NodeID/1 -> set_NMT_state/2
  set_NMT_state/1 -> CAN Write/1

== system ExoskeletonControlModel/DataProcessing/Homing_State_Machine/Homing_m1/HOMING.ST3_set_home_mode/receive_PDO2_m1 ==
  mode : Inport
  Bus Selector : BusSelector  OutputSignals=mode_m1,interpolation_period_m1
  CAN Write : speedgoatlib_IO614/CAN/CAN Write  id=1  sampleTime=-1  portSelection=3  messageType=CAN  enaStatusPort=off  protl=IO614  ptIdx=2  isFDMod=0
  set_mode : canmsglib/CAN Pack  MsgList=(none)  MsgName=CAN Msg  MsgIDType=Standard (11-bit identifier)  MsgIdentifier=hex2dec('301')  MsgLength=2  Remote=off  ApplyMinMax=off  BusOutput=off  SignalInfo={ 'mode', '0', '8', 'LE', 'unsigned', 'Standard', '0', '1', '0', '-Inf', 'Inf'; 'interpolation time period', '8', '8', 'LE', 'unsigned', 'Standard', '0', '1', '0', '-Inf', 'Inf' }
      settings: DataFormat=manually specified signals
  wires:
  set_mode/1 -> CAN Write/1
  mode/1 -> Bus Selector/1
  Bus Selector/1 -> set_mode/1  "<mode_m1>"
  Bus Selector/2 -> set_mode/2  "<interpolation_period_m1>"

== system ExoskeletonControlModel/DataProcessing/Homing_State_Machine/Homing_m1/HOMING.ST4_shutdown/receive_PDO1_m1 ==
  controlword : Inport
  CAN Write : speedgoatlib_IO614/CAN/CAN Write  id=1  sampleTime=-1  portSelection=3  messageType=CAN  enaStatusPort=off  protl=IO614  ptIdx=2  isFDMod=0
  set_controlword : canmsglib/CAN Pack  MsgList=(none)  MsgName=CAN Msg  MsgIDType=Standard (11-bit identifier)  MsgIdentifier=hex2dec('201')  MsgLength=2  Remote=off  ApplyMinMax=off  BusOutput=off  SignalInfo={ 'controlword', '0', '16', 'LE', 'unsigned', 'Standard', '0', '1', '0', '-Inf', 'Inf' }
      settings: DataFormat=manually specified signals
  wires:
  controlword/1 -> set_controlword/1
  set_controlword/1 -> CAN Write/1

== system ExoskeletonControlModel/DataProcessing/Homing_State_Machine/Homing_m1/HOMING.ST5_Switch_on_and_Enable_Operation/receive_PDO1_m1 ==
  controlword : Inport
  CAN Write : speedgoatlib_IO614/CAN/CAN Write  id=1  sampleTime=-1  portSelection=3  messageType=CAN  enaStatusPort=off  protl=IO614  ptIdx=2  isFDMod=0
  set_controlword : canmsglib/CAN Pack  MsgList=(none)  MsgName=CAN Msg  MsgIDType=Standard (11-bit identifier)  MsgIdentifier=hex2dec('201')  MsgLength=2  Remote=off  ApplyMinMax=off  BusOutput=off  SignalInfo={ 'controlword', '0', '16', 'LE', 'unsigned', 'Standard', '0', '1', '0', '-Inf', 'Inf' }
      settings: DataFormat=manually specified signals
  wires:
  controlword/1 -> set_controlword/1
  set_controlword/1 -> CAN Write/1

== system ExoskeletonControlModel/DataProcessing/Homing_State_Machine/Homing_m1/HOMING.ST8_start_homing/receive_PDO1_m1 ==
  controlword : Inport
  CAN Write : speedgoatlib_IO614/CAN/CAN Write  id=1  sampleTime=-1  portSelection=3  messageType=CAN  enaStatusPort=off  protl=IO614  ptIdx=2  isFDMod=0
  set_controlword : canmsglib/CAN Pack  MsgList=(none)  MsgName=CAN Msg  MsgIDType=Standard (11-bit identifier)  MsgIdentifier=hex2dec('201')  MsgLength=2  Remote=off  ApplyMinMax=off  BusOutput=off  SignalInfo={ 'controlword', '0', '16', 'LE', 'unsigned', 'Standard', '0', '1', '0', '-Inf', 'Inf' }
      settings: DataFormat=manually specified signals
  wires:
  controlword/1 -> set_controlword/1
  set_controlword/1 -> CAN Write/1

== system ExoskeletonControlModel/DataProcessing/Homing_State_Machine/Homing_m1/HOMING.ST9_stop_homing/receive_PDO1_m1 ==
  controlword : Inport
  CAN Write : speedgoatlib_IO614/CAN/CAN Write  id=1  sampleTime=-1  portSelection=3  messageType=CAN  enaStatusPort=off  protl=IO614  ptIdx=2  isFDMod=0
  set_controlword : canmsglib/CAN Pack  MsgList=(none)  MsgName=CAN Msg  MsgIDType=Standard (11-bit identifier)  MsgIdentifier=hex2dec('201')  MsgLength=2  Remote=off  ApplyMinMax=off  BusOutput=off  SignalInfo={ 'controlword', '0', '16', 'LE', 'unsigned', 'Standard', '0', '1', '0', '-Inf', 'Inf' }
      settings: DataFormat=manually specified signals
  wires:
  controlword/1 -> set_controlword/1
  set_controlword/1 -> CAN Write/1

== system ExoskeletonControlModel/DataProcessing/Homing_State_Machine/Homing_m2/FAULT.Fault_reset/receive_PDO1_m1 ==
  controlword : Inport
  CAN Write : speedgoatlib_IO614/CAN/CAN Write  id=1  sampleTime=-1  portSelection=3  messageType=CAN  enaStatusPort=off  protl=IO614  ptIdx=2  isFDMod=0
  set_controlword : canmsglib/CAN Pack  MsgList=(none)  MsgName=CAN Msg  MsgIDType=Standard (11-bit identifier)  MsgIdentifier=hex2dec('202')  MsgLength=2  Remote=off  ApplyMinMax=off  BusOutput=off  SignalInfo={ 'controlword', '0', '16', 'LE', 'unsigned', 'Standard', '0', '1', '0', '-Inf', 'Inf' }
      settings: DataFormat=manually specified signals
  wires:
  controlword/1 -> set_controlword/1
  set_controlword/1 -> CAN Write/1

== system ExoskeletonControlModel/DataProcessing/Homing_State_Machine/Homing_m2/FAULT.ST4_shutdown/receive_PDO1_m1 ==
  controlword : Inport
  CAN Write : speedgoatlib_IO614/CAN/CAN Write  id=1  sampleTime=-1  portSelection=3  messageType=CAN  enaStatusPort=off  protl=IO614  ptIdx=2  isFDMod=0
  set_controlword : canmsglib/CAN Pack  MsgList=(none)  MsgName=CAN Msg  MsgIDType=Standard (11-bit identifier)  MsgIdentifier=hex2dec('202')  MsgLength=2  Remote=off  ApplyMinMax=off  BusOutput=off  SignalInfo={ 'controlword', '0', '16', 'LE', 'unsigned', 'Standard', '0', '1', '0', '-Inf', 'Inf' }
      settings: DataFormat=manually specified signals
  wires:
  controlword/1 -> set_controlword/1
  set_controlword/1 -> CAN Write/1

== system ExoskeletonControlModel/DataProcessing/Homing_State_Machine/Homing_m2/HOMING.ST10_set_PPM/receive_PDO2_m1 ==
  mode : Inport
  Bus Selector : BusSelector  OutputSignals=mode_m1,interpolation_period_m1
  CAN Write : speedgoatlib_IO614/CAN/CAN Write  id=1  sampleTime=-1  portSelection=3  messageType=CAN  enaStatusPort=off  protl=IO614  ptIdx=2  isFDMod=0
  set_mode : canmsglib/CAN Pack  MsgList=(none)  MsgName=CAN Msg  MsgIDType=Standard (11-bit identifier)  MsgIdentifier=hex2dec('302')  MsgLength=2  Remote=off  ApplyMinMax=off  BusOutput=off  SignalInfo={ 'mode', '0', '8', 'LE', 'unsigned', 'Standard', '0', '1', '0', '-Inf', 'Inf'; 'interpolation time period', '8', '8', 'LE', 'unsigned', 'Standard', '0', '1', '0', '-Inf', 'Inf' }
      settings: DataFormat=manually specified signals
  wires:
  set_mode/1 -> CAN Write/1
  mode/1 -> Bus Selector/1
  Bus Selector/1 -> set_mode/1  "<mode_m1>"
  Bus Selector/2 -> set_mode/2  "<interpolation_period_m1>"

== system ExoskeletonControlModel/DataProcessing/Homing_State_Machine/Homing_m2/HOMING.ST11_shutdown1/receive_PDO1_m1 ==
  controlword : Inport
  CAN Write : speedgoatlib_IO614/CAN/CAN Write  id=1  sampleTime=-1  portSelection=3  messageType=CAN  enaStatusPort=off  protl=IO614  ptIdx=2  isFDMod=0
  set_controlword : canmsglib/CAN Pack  MsgList=(none)  MsgName=CAN Msg  MsgIDType=Standard (11-bit identifier)  MsgIdentifier=hex2dec('202')  MsgLength=2  Remote=off  ApplyMinMax=off  BusOutput=off  SignalInfo={ 'controlword', '0', '16', 'LE', 'unsigned', 'Standard', '0', '1', '0', '-Inf', 'Inf' }
      settings: DataFormat=manually specified signals
  wires:
  controlword/1 -> set_controlword/1
  set_controlword/1 -> CAN Write/1

== system ExoskeletonControlModel/DataProcessing/Homing_State_Machine/Homing_m2/HOMING.ST12_Switch_on_and_Enable_Operation/receive_PDO1_m1 ==
  controlword : Inport
  CAN Write : speedgoatlib_IO614/CAN/CAN Write  id=1  sampleTime=-1  portSelection=3  messageType=CAN  enaStatusPort=off  protl=IO614  ptIdx=2  isFDMod=0
  set_controlword : canmsglib/CAN Pack  MsgList=(none)  MsgName=CAN Msg  MsgIDType=Standard (11-bit identifier)  MsgIdentifier=hex2dec('202')  MsgLength=2  Remote=off  ApplyMinMax=off  BusOutput=off  SignalInfo={ 'controlword', '0', '16', 'LE', 'unsigned', 'Standard', '0', '1', '0', '-Inf', 'Inf' }
      settings: DataFormat=manually specified signals
  wires:
  controlword/1 -> set_controlword/1
  set_controlword/1 -> CAN Write/1

== system ExoskeletonControlModel/DataProcessing/Homing_State_Machine/Homing_m2/HOMING.ST13_send_target_pos/receive_PDO3_m1 ==
  target_pos : Inport
  CAN Write : speedgoatlib_IO614/CAN/CAN Write  id=1  sampleTime=-1  portSelection=3  messageType=CAN  enaStatusPort=off  protl=IO614  ptIdx=2  isFDMod=0
  set_position : canmsglib/CAN Pack  MsgList=(none)  MsgName=CAN Msg  MsgIDType=Standard (11-bit identifier)  MsgIdentifier=hex2dec('402')  MsgLength=4  Remote=off  ApplyMinMax=off  BusOutput=off  SignalInfo={ 'target position', '0', '32', 'LE', 'signed', 'Standard', '0', '1', '0', '-Inf', 'Inf' }
      settings: DataFormat=manually specified signals
  wires:
  target_pos/1 -> set_position/1
  set_position/1 -> CAN Write/1

== system ExoskeletonControlModel/DataProcessing/Homing_State_Machine/Homing_m2/HOMING.ST14_Abs_ref_start_immediatly/receive_PDO1_m1 ==
  controlword : Inport
  CAN Write : speedgoatlib_IO614/CAN/CAN Write  id=1  sampleTime=-1  portSelection=3  messageType=CAN  enaStatusPort=off  protl=IO614  ptIdx=2  isFDMod=0
  set_controlword : canmsglib/CAN Pack  MsgList=(none)  MsgName=CAN Msg  MsgIDType=Standard (11-bit identifier)  MsgIdentifier=hex2dec('202')  MsgLength=2  Remote=off  ApplyMinMax=off  BusOutput=off  SignalInfo={ 'controlword', '0', '16', 'LE', 'unsigned', 'Standard', '0', '1', '0', '-Inf', 'Inf' }
      settings: DataFormat=manually specified signals
  wires:
  controlword/1 -> set_controlword/1
  set_controlword/1 -> CAN Write/1

== system ExoskeletonControlModel/DataProcessing/Homing_State_Machine/Homing_m2/HOMING.ST15_set_home_mode/receive_PDO2_m1 ==
  mode : Inport
  Bus Selector : BusSelector  OutputSignals=mode_m1,interpolation_period_m1
  CAN Write : speedgoatlib_IO614/CAN/CAN Write  id=1  sampleTime=-1  portSelection=3  messageType=CAN  enaStatusPort=off  protl=IO614  ptIdx=2  isFDMod=0
  set_mode : canmsglib/CAN Pack  MsgList=(none)  MsgName=CAN Msg  MsgIDType=Standard (11-bit identifier)  MsgIdentifier=hex2dec('302')  MsgLength=2  Remote=off  ApplyMinMax=off  BusOutput=off  SignalInfo={ 'mode', '0', '8', 'LE', 'unsigned', 'Standard', '0', '1', '0', '-Inf', 'Inf'; 'interpolation time period', '8', '8', 'LE', 'unsigned', 'Standard', '0', '1', '0', '-Inf', 'Inf' }
      settings: DataFormat=manually specified signals
  wires:
  set_mode/1 -> CAN Write/1
  mode/1 -> Bus Selector/1
  Bus Selector/1 -> set_mode/1  "<mode_m1>"
  Bus Selector/2 -> set_mode/2  "<interpolation_period_m1>"

== system ExoskeletonControlModel/DataProcessing/Homing_State_Machine/Homing_m2/HOMING.ST3_set_home_mode/receive_PDO2_m1 ==
  mode : Inport
  Bus Selector : BusSelector  OutputSignals=mode_m1,interpolation_period_m1
  CAN Write : speedgoatlib_IO614/CAN/CAN Write  id=1  sampleTime=-1  portSelection=3  messageType=CAN  enaStatusPort=off  protl=IO614  ptIdx=2  isFDMod=0
  set_mode : canmsglib/CAN Pack  MsgList=(none)  MsgName=CAN Msg  MsgIDType=Standard (11-bit identifier)  MsgIdentifier=hex2dec('302')  MsgLength=2  Remote=off  ApplyMinMax=off  BusOutput=off  SignalInfo={ 'mode', '0', '8', 'LE', 'unsigned', 'Standard', '0', '1', '0', '-Inf', 'Inf'; 'interpolation time period', '8', '8', 'LE', 'unsigned', 'Standard', '0', '1', '0', '-Inf', 'Inf' }
      settings: DataFormat=manually specified signals
  wires:
  set_mode/1 -> CAN Write/1
  mode/1 -> Bus Selector/1
  Bus Selector/1 -> set_mode/1  "<mode_m1>"
  Bus Selector/2 -> set_mode/2  "<interpolation_period_m1>"

== system ExoskeletonControlModel/DataProcessing/Homing_State_Machine/Homing_m2/HOMING.ST4_shutdown/receive_PDO1_m1 ==
  controlword : Inport
  CAN Write : speedgoatlib_IO614/CAN/CAN Write  id=1  sampleTime=-1  portSelection=3  messageType=CAN  enaStatusPort=off  protl=IO614  ptIdx=2  isFDMod=0
  set_controlword : canmsglib/CAN Pack  MsgList=(none)  MsgName=CAN Msg  MsgIDType=Standard (11-bit identifier)  MsgIdentifier=hex2dec('202')  MsgLength=2  Remote=off  ApplyMinMax=off  BusOutput=off  SignalInfo={ 'controlword', '0', '16', 'LE', 'unsigned', 'Standard', '0', '1', '0', '-Inf', 'Inf' }
      settings: DataFormat=manually specified signals
  wires:
  controlword/1 -> set_controlword/1
  set_controlword/1 -> CAN Write/1

== system ExoskeletonControlModel/DataProcessing/Homing_State_Machine/Homing_m2/HOMING.ST5_Switch_on_and_Enable_Operation/receive_PDO1_m1 ==
  controlword : Inport
  CAN Write : speedgoatlib_IO614/CAN/CAN Write  id=1  sampleTime=-1  portSelection=3  messageType=CAN  enaStatusPort=off  protl=IO614  ptIdx=2  isFDMod=0
  set_controlword : canmsglib/CAN Pack  MsgList=(none)  MsgName=CAN Msg  MsgIDType=Standard (11-bit identifier)  MsgIdentifier=hex2dec('202')  MsgLength=2  Remote=off  ApplyMinMax=off  BusOutput=off  SignalInfo={ 'controlword', '0', '16', 'LE', 'unsigned', 'Standard', '0', '1', '0', '-Inf', 'Inf' }
      settings: DataFormat=manually specified signals
  wires:
  controlword/1 -> set_controlword/1
  set_controlword/1 -> CAN Write/1

== system ExoskeletonControlModel/DataProcessing/Homing_State_Machine/Homing_m2/HOMING.ST8_start_homing/receive_PDO1_m1 ==
  controlword : Inport
  CAN Write : speedgoatlib_IO614/CAN/CAN Write  id=1  sampleTime=-1  portSelection=3  messageType=CAN  enaStatusPort=off  protl=IO614  ptIdx=2  isFDMod=0
  set_controlword : canmsglib/CAN Pack  MsgList=(none)  MsgName=CAN Msg  MsgIDType=Standard (11-bit identifier)  MsgIdentifier=hex2dec('202')  MsgLength=2  Remote=off  ApplyMinMax=off  BusOutput=off  SignalInfo={ 'controlword', '0', '16', 'LE', 'unsigned', 'Standard', '0', '1', '0', '-Inf', 'Inf' }
      settings: DataFormat=manually specified signals
  wires:
  controlword/1 -> set_controlword/1
  set_controlword/1 -> CAN Write/1

== system ExoskeletonControlModel/DataProcessing/Homing_State_Machine/Homing_m2/HOMING.ST9_stop_homing/receive_PDO1_m1 ==
  controlword : Inport
  CAN Write : speedgoatlib_IO614/CAN/CAN Write  id=1  sampleTime=-1  portSelection=3  messageType=CAN  enaStatusPort=off  protl=IO614  ptIdx=2  isFDMod=0
  set_controlword : canmsglib/CAN Pack  MsgList=(none)  MsgName=CAN Msg  MsgIDType=Standard (11-bit identifier)  MsgIdentifier=hex2dec('202')  MsgLength=2  Remote=off  ApplyMinMax=off  BusOutput=off  SignalInfo={ 'controlword', '0', '16', 'LE', 'unsigned', 'Standard', '0', '1', '0', '-Inf', 'Inf' }
      settings: DataFormat=manually specified signals
  wires:
  controlword/1 -> set_controlword/1
  set_controlword/1 -> CAN Write/1

== system ExoskeletonControlModel/DataProcessing/Homing_State_Machine/Homing_m3/FAULT.Fault_reset/receive_PDO1_m1 ==
  controlword : Inport
  CAN Write : speedgoatlib_IO614/CAN/CAN Write  id=1  sampleTime=-1  portSelection=4  messageType=CAN  enaStatusPort=off  protl=IO614  ptIdx=3  isFDMod=0
  set_controlword : canmsglib/CAN Pack  MsgList=(none)  MsgName=CAN Msg  MsgIDType=Standard (11-bit identifier)  MsgIdentifier=hex2dec('201')  MsgLength=2  Remote=off  ApplyMinMax=off  BusOutput=off  SignalInfo={ 'controlword', '0', '16', 'LE', 'unsigned', 'Standard', '0', '1', '0', '-Inf', 'Inf' }
      settings: DataFormat=manually specified signals
  wires:
  controlword/1 -> set_controlword/1
  set_controlword/1 -> CAN Write/1

== system ExoskeletonControlModel/DataProcessing/Homing_State_Machine/Homing_m3/FAULT.ST4_shutdown/receive_PDO1_m1 ==
  controlword : Inport
  CAN Write : speedgoatlib_IO614/CAN/CAN Write  id=1  sampleTime=-1  portSelection=4  messageType=CAN  enaStatusPort=off  protl=IO614  ptIdx=3  isFDMod=0
  set_controlword : canmsglib/CAN Pack  MsgList=(none)  MsgName=CAN Msg  MsgIDType=Standard (11-bit identifier)  MsgIdentifier=hex2dec('201')  MsgLength=2  Remote=off  ApplyMinMax=off  BusOutput=off  SignalInfo={ 'controlword', '0', '16', 'LE', 'unsigned', 'Standard', '0', '1', '0', '-Inf', 'Inf' }
      settings: DataFormat=manually specified signals
  wires:
  controlword/1 -> set_controlword/1
  set_controlword/1 -> CAN Write/1

== system ExoskeletonControlModel/DataProcessing/Homing_State_Machine/Homing_m3/HOMING.ST10_set_PPM/receive_PDO2_m1 ==
  mode : Inport
  Bus Selector : BusSelector  OutputSignals=mode_m1,interpolation_period_m1
  CAN Write : speedgoatlib_IO614/CAN/CAN Write  id=1  sampleTime=-1  portSelection=4  messageType=CAN  enaStatusPort=off  protl=IO614  ptIdx=3  isFDMod=0
  set_mode : canmsglib/CAN Pack  MsgList=(none)  MsgName=CAN Msg  MsgIDType=Standard (11-bit identifier)  MsgIdentifier=hex2dec('301')  MsgLength=2  Remote=off  ApplyMinMax=off  BusOutput=off  SignalInfo={ 'mode', '0', '8', 'LE', 'unsigned', 'Standard', '0', '1', '0', '-Inf', 'Inf'; 'interpolation time period', '8', '8', 'LE', 'unsigned', 'Standard', '0', '1', '0', '-Inf', 'Inf' }
      settings: DataFormat=manually specified signals
  wires:
  set_mode/1 -> CAN Write/1
  mode/1 -> Bus Selector/1
  Bus Selector/1 -> set_mode/1  "<mode_m1>"
  Bus Selector/2 -> set_mode/2  "<interpolation_period_m1>"

== system ExoskeletonControlModel/DataProcessing/Homing_State_Machine/Homing_m3/HOMING.ST11_shutdown1/receive_PDO1_m1 ==
  controlword : Inport
  CAN Write : speedgoatlib_IO614/CAN/CAN Write  id=1  sampleTime=-1  portSelection=4  messageType=CAN  enaStatusPort=off  protl=IO614  ptIdx=3  isFDMod=0
  set_controlword : canmsglib/CAN Pack  MsgList=(none)  MsgName=CAN Msg  MsgIDType=Standard (11-bit identifier)  MsgIdentifier=hex2dec('201')  MsgLength=2  Remote=off  ApplyMinMax=off  BusOutput=off  SignalInfo={ 'controlword', '0', '16', 'LE', 'unsigned', 'Standard', '0', '1', '0', '-Inf', 'Inf' }
      settings: DataFormat=manually specified signals
  wires:
  controlword/1 -> set_controlword/1
  set_controlword/1 -> CAN Write/1

== system ExoskeletonControlModel/DataProcessing/Homing_State_Machine/Homing_m3/HOMING.ST12_Switch_on_and_Enable_Operation/receive_PDO1_m1 ==
  controlword : Inport
  CAN Write : speedgoatlib_IO614/CAN/CAN Write  id=1  sampleTime=-1  portSelection=4  messageType=CAN  enaStatusPort=off  protl=IO614  ptIdx=3  isFDMod=0
  set_controlword : canmsglib/CAN Pack  MsgList=(none)  MsgName=CAN Msg  MsgIDType=Standard (11-bit identifier)  MsgIdentifier=hex2dec('201')  MsgLength=2  Remote=off  ApplyMinMax=off  BusOutput=off  SignalInfo={ 'controlword', '0', '16', 'LE', 'unsigned', 'Standard', '0', '1', '0', '-Inf', 'Inf' }
      settings: DataFormat=manually specified signals
  wires:
  controlword/1 -> set_controlword/1
  set_controlword/1 -> CAN Write/1

== system ExoskeletonControlModel/DataProcessing/Homing_State_Machine/Homing_m3/HOMING.ST13_send_target_pos/receive_PDO3_m1 ==
  target_pos : Inport
  CAN Write : speedgoatlib_IO614/CAN/CAN Write  id=1  sampleTime=-1  portSelection=4  messageType=CAN  enaStatusPort=off  protl=IO614  ptIdx=3  isFDMod=0
  set_position : canmsglib/CAN Pack  MsgList=(none)  MsgName=CAN Msg  MsgIDType=Standard (11-bit identifier)  MsgIdentifier=hex2dec('401')  MsgLength=4  Remote=off  ApplyMinMax=off  BusOutput=off  SignalInfo={ 'target position', '0', '32', 'LE', 'signed', 'Standard', '0', '1', '0', '-Inf', 'Inf' }
      settings: DataFormat=manually specified signals
  wires:
  target_pos/1 -> set_position/1
  set_position/1 -> CAN Write/1

== system ExoskeletonControlModel/DataProcessing/Homing_State_Machine/Homing_m3/HOMING.ST14_Abs_ref_start_immediatly/receive_PDO1_m1 ==
  controlword : Inport
  CAN Write : speedgoatlib_IO614/CAN/CAN Write  id=1  sampleTime=-1  portSelection=4  messageType=CAN  enaStatusPort=off  protl=IO614  ptIdx=3  isFDMod=0
  set_controlword : canmsglib/CAN Pack  MsgList=(none)  MsgName=CAN Msg  MsgIDType=Standard (11-bit identifier)  MsgIdentifier=hex2dec('201')  MsgLength=2  Remote=off  ApplyMinMax=off  BusOutput=off  SignalInfo={ 'controlword', '0', '16', 'LE', 'unsigned', 'Standard', '0', '1', '0', '-Inf', 'Inf' }
      settings: DataFormat=manually specified signals
  wires:
  controlword/1 -> set_controlword/1
  set_controlword/1 -> CAN Write/1
